simulink model "prelab2_DCmotor"  (R2019b)
settings: Solver=FixedStepAuto  StartTime=0.0  StopTime=10.0  RelTol=1e-3
values from neighbouring files (symbols this model uses):
  clock_c = 0.26    [workspace.mat]
  k = 14.4844    [workspace.mat]
  p = 190    [workspace.mat]
  tau = 0.191    [LabWork2.m]    (also in workspace.mat)
  z = 48    [workspace.mat]
libraries: simulink x2
settings Model: Creator=MSI  LastModifiedBy=MSI

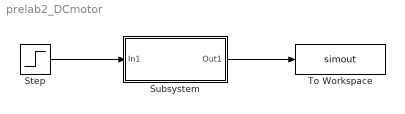
== system prelab2_DCmotor ==
  Step : Step  Time=0  After=9  SampleTime=0
  Subsystem : Subsystem
  To Workspace : ToWorkspace  VariableName=simout  SaveFormat=Timeseries  SampleTime=-1
  wires:
  Step/1 -> Subsystem/1(In1)
  Subsystem/1(Out1) -> To Workspace/1

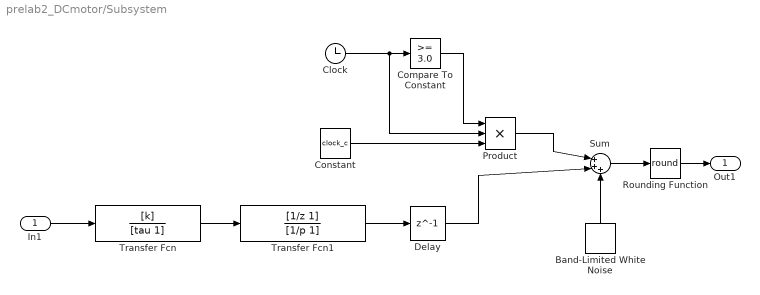
== system prelab2_DCmotor/Subsystem ==
  In1 : Inport
  Band-Limited White Noise : simulink/Sources/Band-Limited White Noise  Cov=[0.002]  Ts=0.01  seed=[23341]
  Clock : Clock
  Compare To Constant : simulink/Logic and Bit Operations/Compare To Constant  relop=>=  const=3.0  OutDataTypeStr=uint8
  Constant : Constant  Value=clock_c
  Delay : Delay  DelayLength=1
  Product : Product  Inputs=3
  Rounding Function : Rounding  Operator=round
  Sum : Sum  Inputs=|+++
  Transfer Fcn : TransferFcn  Numerator=[k]  Denominator=[tau 1]
  Transfer Fcn1 : TransferFcn  Numerator=[1/z 1]  Denominator=[1/p 1]
  Out1 : Outport
  wires:
  Transfer Fcn/1 -> Transfer Fcn1/1
  In1/1 -> Transfer Fcn/1
  Clock/1 -> Product/2, Compare To Constant/1
  Rounding Function/1 -> Out1/1
  Sum/1 -> Rounding Function/1
  Product/1 -> Sum/1
  Transfer Fcn1/1 -> Delay/1
  Band-Limited White Noise/1 -> Sum/3
  Delay/1 -> Sum/2
  Compare To Constant/1 -> Product/1
  Constant/1 -> Product/3
